simulink model "CVCA_TRAINING_21"  (R2021a)
settings: Solver=ode113  StartTime=0.0  StopTime=20  RelTol=1e-3
undefined symbols (not defined in the file or in its folder): Discrete, linsys1, Time
libraries: spsThreePhaseVIMeasurementLib x46, spsThreePhasePISectionLineLib x20, simulink x12, spsThreePhaseSeriesRLCLoadLib x12, spsThreePhaseBreakerLib x6, spsThreePhaseTransformerTwoWindingsLib x5, ctrlSharedLib x3, spsSynchronousMachinepuStandardLib x3, spsThreePhaseParallelRLCLoadLib x3, spsExcitationSystemLib x3, spsGenericPowerSystemStabilizerLib x3, spsHydraulicTurbineandGovernorLib x3
(part 1 of 2)
settings Model: Creator=root  LastModifiedBy=suman
settings DataIOCC: SaveFormat=Array  SaveOutput=off  SignalLogging=off  DSMLogging=off  SaveTime=off  ReturnWorkspaceOutputs=off
settings DebuggingCC: SFMachineParentedDataDiag=warning  ArithmeticOperatorsInVariantConditions=warning
settings SFSimCC: CustomCodeUndefinedFunction=UseInterfaceOnly

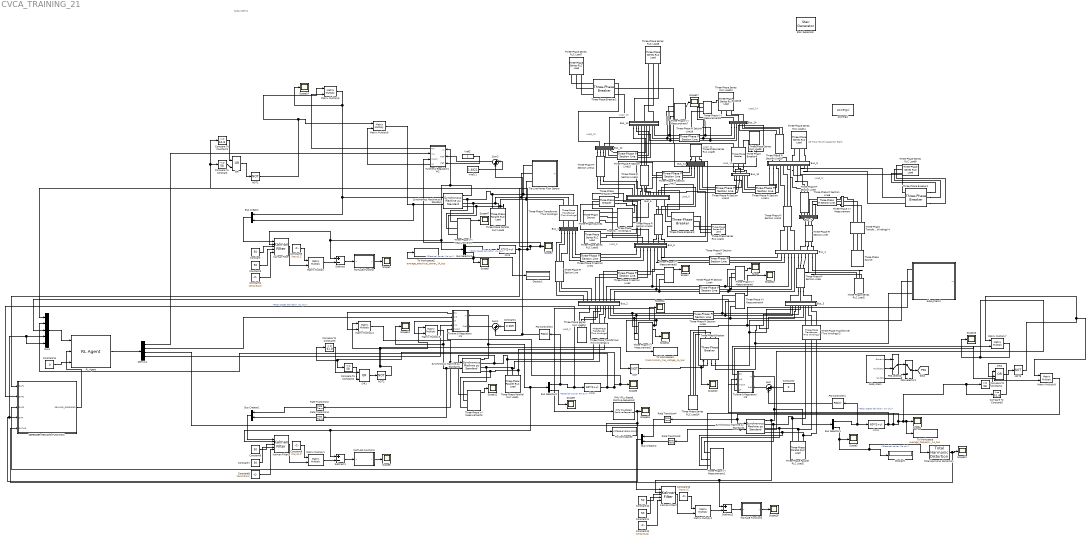
== system CVCA_TRAINING_21 ==
  note: Subsystem1
  note: Load_14
  note: Load_5
  note: Load_9
  note: Load_10
  note: 25 MVar Shunt
      | Capacitor Bank
  note: Load_6
  note: Load_11
  note: Load_13
  note: Load_12
  note: Load_2
  Bus Creator : BusCreator  Inputs=2
  Bus Creator1 : BusCreator  Inputs=2
  Bus Creator2 : BusCreator  Inputs=2
  Bus Selector1 : BusSelector  OutputSignals="Mechanical.Rotor speed deviation  dw (pu),Mechanical.Electrical power  Pe (pu)"
  Bus Selector2 : BusSelector  OutputSignals="Mechanical.Rotor speed deviation  dw (pu),Mechanical.Electrical power  Pe (pu)"
  Bus Selector3 : BusSelector  OutputSignals="Mechanical.Rotor speed deviation  dw (pu),Mechanical.Electrical power  Pe (pu)"
  Bus_1 : Subsystem
  Bus_10 : Subsystem
  Bus_11 : Subsystem
  Bus_12 : Subsystem
  Bus_13 : Subsystem
  Bus_14 : Subsystem
  Bus_2 : Subsystem
  Bus_3 : Subsystem
  Bus_4 : Subsystem
  Bus_5 : Subsystem
  Bus_6 : Subsystem
  Bus_7 : Subsystem
  Bus_9 : Subsystem
  Compare To Constant : simulink/Logic and Bit Operations/Compare To Constant  relop=<=  const=58  OutDataTypeStr=boolean
  Compare To Constant1 : simulink/Logic and Bit Operations/Compare To Constant  relop=>=  const=61.8  OutDataTypeStr=boolean
  Compare To Constant2 : simulink/Logic and Bit Operations/Compare To Constant  relop=<=  const=58  OutDataTypeStr=boolean
  Compare To Constant3 : simulink/Logic and Bit Operations/Compare To Constant  relop=>=  const=61.8  OutDataTypeStr=boolean
  Compare To Constant4 : simulink/Logic and Bit Operations/Compare To Constant  relop=<=  const=58  OutDataTypeStr=boolean
  Compare To Constant5 : simulink/Logic and Bit Operations/Compare To Constant  relop=>=  const=61.8  OutDataTypeStr=boolean
  Constant{,3,6..7,10..11} (6 alike) : Constant  Value=50
  Constant1 : Constant  Value=2.009
  Constant12 : Constant  Value=zeros(8,24)
  Constant13 : Constant  Value=linsys1.C
  Constant14 : Constant  Value=0
  Constant2 : Constant  Value=0
  Constant4 : Constant  Value=zeros(8,24)
  Constant5 : Constant  Value=linsys1.C
  Constant8 : Constant  Value=zeros(8,24)
  Constant9 : Constant  Value=linsys1.C
  DEFENDER REWARD FUNCTION : MATLAB Function  TreatAsAtomicUnit=on
  Demux1 : Demux
  Display1 : Display
  Display5 : Display
  Fcn1 : Fcn  Expr=60*(1+u)
  Fcn2 : Fcn  Expr=60*(1+u)
  Fcn3 : Fcn  Expr=60*(1+u)
  Kalman Filter : ctrlSharedLib/Kalman Filter  TimeDomain=Discrete-Time  UseCurrentEstimator=on  ModelSource=Individual A, B, C, D matrices  ModelSourceVariable=ss(0.95,1,1,0,1)  A=linsys1.A  B=linsys1.B  C=linsys1.C  D=linsys1.D  NumberOfStates=1  NumberOfInputs=1  NumberOfOutputs=1  InitialEstimateSource=Dialog  X0=0  P0=10  UseK=off  UseGH=off  NumberOfProcessNoiseInputs=1  G=1  TimeInvariantG=on  H=0  TimeInvariantH=on  Q=0.05  TimeInvariantQ=off  R=1  TimeInvariantR=off  N=0  TimeInvariantN=off  AddInputPort=on  AddEnablePort=off  OutputEstimatedY=off  OutputP=off  Ts=-1
  Kalman Filter1 : ctrlSharedLib/Kalman Filter  TimeDomain=Discrete-Time  UseCurrentEstimator=on  ModelSource=Individual A, B, C, D matrices  ModelSourceVariable=ss(0.95,1,1,0,1)  A=linsys1.A  B=linsys1.B  C=linsys1.C  D=linsys1.D  NumberOfStates=1  NumberOfInputs=1  NumberOfOutputs=1  InitialEstimateSource=Dialog  X0=0  P0=10  UseK=off  UseGH=off  NumberOfProcessNoiseInputs=1  G=1  TimeInvariantG=on  H=0  TimeInvariantH=on  Q=0.05  TimeInvariantQ=off  R=1  TimeInvariantR=off  N=0  TimeInvariantN=off  AddInputPort=on  AddEnablePort=off  OutputEstimatedY=off  OutputP=off  Ts=-1
  Kalman Filter2 : ctrlSharedLib/Kalman Filter  TimeDomain=Discrete-Time  UseCurrentEstimator=on  ModelSource=Individual A, B, C, D matrices  ModelSourceVariable=ss(0.95,1,1,0,1)  A=linsys1.A  B=linsys1.B  C=linsys1.C  D=linsys1.D  NumberOfStates=1  NumberOfInputs=1  NumberOfOutputs=1  InitialEstimateSource=Dialog  X0=0  P0=10  UseK=off  UseGH=off  NumberOfProcessNoiseInputs=1  G=1  TimeInvariantG=on  H=0  TimeInvariantH=on  Q=0.05  TimeInvariantQ=off  R=1  TimeInvariantR=off  N=0  TimeInvariantN=off  AddInputPort=on  AddEnablePort=off  OutputEstimatedY=off  OutputP=off  Ts=-1
  MATLAB Function : MATLAB Function  TreatAsAtomicUnit=on
  MATLAB Function1 : MATLAB Function  TreatAsAtomicUnit=on
  MATLAB Function2 : MATLAB Function  TreatAsAtomicUnit=on
  Matrix Multiply{,1..8} (9 alike) : Product  Multiplication=Matrix(*)
  Mux1 : Mux  Inputs=5
  NOT{,1..3} (4 alike) : Logic  Operator=NOT  IconShape=distinctive  AllPortsSameDT=off  OutDataTypeStr=boolean
  OR : Logic  Operator=OR  IconShape=distinctive  AllPortsSameDT=off  OutDataTypeStr=boolean
  OR1 : Logic  Operator=OR  IconShape=distinctive  AllPortsSameDT=off  OutDataTypeStr=boolean
  OR2 : Logic  Operator=OR  IconShape=distinctive  AllPortsSameDT=off  OutDataTypeStr=boolean
  PID Controller1 : slpidlib/PID Controller  Controller=PID  Form=Parallel  TimeDomain=Discrete-time  UseExternalTs=off  SampleTime=-1  IntegratorMethod=Forward Euler  FilterMethod=Forward Euler  ControllerParametersSource=internal  P=-0.020868  I=-0.0020766  D=0  UseFilter=on  N=100  TunerSelectOption=Frequency Response Based  InitialConditionSource=internal  InitialConditionForIntegrator=0  InitialConditionForFilter=0  DifferentiatorICPrevScaledInput=0  ExternalReset=none  TrackingMode=off  Kt=1  LimitOutput=off  SatLimitsSource=internal  UpperSaturationLimit=inf  LowerSaturationLimit=-inf  LinearizeAsGain=on  AntiWindupMode=none  Kb=1  POutMin=[]  POutMax=[]  IOutMin=[]  IOutMax=[]  DOutMin=[]  DOutMax=[]  NOutMin=[]  NOutMax=[]  SumOutMin=[]  SumOutMax=[]  SaturationOutMin=[]  SaturationOutMax=[]  PParamMin=[]  PParamMax=[]  IParamMin=[]  IParamMax=[]  DParamMin=[]  DParamMax=[]  NParamMin=[]  NParamMax=[]  KbParamMin=[]  KbParamMax=[]  KtParamMin=[]  KtParamMax=[]  KbOutMin=[]  KbOutMax=[]  KtOutMin=[]  KtOutMax=[]  IntegratorOutMin=[]  IntegratorOutMax=[]  FilterOutMin=[]  FilterOutMax=[]  SumI1OutMin=[]  SumI1OutMax=[]  SumI2OutMin=[]  SumI2OutMax=[]  SumI3OutMin=[]  SumI3OutMax=[]  SumI4OutMin=[]  SumI4OutMax=[]  SumDOutMin=[]  SumDOutMax=[]  DifferentiatorOutMin=[]  DifferentiatorOutMax=[]  FilterDiffOutCoefMin=[]  FilterDiffOutCoefMax=[]  ReciprocalOutMin=[]  ReciprocalOutMax=[]  SumDenOutMin=[]  SumDenOutMax=[]  SumNumOutMin=[]  SumNumOutMax=[]  DivideOutMin=[]  DivideOutMax=[]  UdiffTsProdOutMin=[]  UdiffTsProdOutMax=[]  NTsProdOutMin=[]  NTsProdOutMax=[]  UintegralTsProdOutMin=[]  UintegralTsProdOutMax=[]  UngainTsProdOutMin=[]  UngainTsProdOutMax=[]  IntegratorContinuousStateAttributes=''  IntegratorStateMustResolveToSignalObject=off  IntegratorRTWStateStorageClass=Auto  FilterContinuousStateAttributes=''  FilterStateMustResolveToSignalObject=off  FilterRTWStateStorageClass=Auto  ParallelPVariant=InternalParameters  IdealPVariant=Disabled  IVariant=InternalParameters  DVariant=InternalParameters  IntegratorVariant=Discrete  SatVariant=Disabled  AWVariant=Passthrough  PCopyVariant=Disabled  TRVariant=Disabled  FdbkBlocksVariant=Forward  IdealPFdbkVariant=Disabled  SatFdbkVariant=Disabled  DerivativeFilterVariant=ForwardEulerFilter  NVariant=InternalParameters  NCopyVariant=Disabled  FilterICVariant=InternalICsFilter  IntegratorICVariant=InternalICs  ExternalResetVariant=Disabled  TRSumVariant=Passthrough  SumFdbkVariant=Disabled  SumVariant=Sum_PID  TsampFilterVariant=InternalTs  TsampNgainVariant=Passthrough  TsampIntegralVariant=Passthrough  ExternalSaturationOutDataTypeStr=Inherit: Same as second input
  PID Controller2 : slpidlib/PID Controller  Controller=PID  Form=Parallel  TimeDomain=Discrete-time  UseExternalTs=off  SampleTime=-1  IntegratorMethod=Forward Euler  FilterMethod=Forward Euler  ControllerParametersSource=internal  P=-0.020868  I=-0.0020766  D=0  UseFilter=on  N=100  TunerSelectOption=Frequency Response Based  InitialConditionSource=internal  InitialConditionForIntegrator=0  InitialConditionForFilter=0  DifferentiatorICPrevScaledInput=0  ExternalReset=none  TrackingMode=off  Kt=1  LimitOutput=off  SatLimitsSource=internal  UpperSaturationLimit=inf  LowerSaturationLimit=-inf  LinearizeAsGain=on  AntiWindupMode=none  Kb=1  POutMin=[]  POutMax=[]  IOutMin=[]  IOutMax=[]  DOutMin=[]  DOutMax=[]  NOutMin=[]  NOutMax=[]  SumOutMin=[]  SumOutMax=[]  SaturationOutMin=[]  SaturationOutMax=[]  PParamMin=[]  PParamMax=[]  IParamMin=[]  IParamMax=[]  DParamMin=[]  DParamMax=[]  NParamMin=[]  NParamMax=[]  KbParamMin=[]  KbParamMax=[]  KtParamMin=[]  KtParamMax=[]  KbOutMin=[]  KbOutMax=[]  KtOutMin=[]  KtOutMax=[]  IntegratorOutMin=[]  IntegratorOutMax=[]  FilterOutMin=[]  FilterOutMax=[]  SumI1OutMin=[]  SumI1OutMax=[]  SumI2OutMin=[]  SumI2OutMax=[]  SumI3OutMin=[]  SumI3OutMax=[]  SumI4OutMin=[]  SumI4OutMax=[]  SumDOutMin=[]  SumDOutMax=[]  DifferentiatorOutMin=[]  DifferentiatorOutMax=[]  FilterDiffOutCoefMin=[]  FilterDiffOutCoefMax=[]  ReciprocalOutMin=[]  ReciprocalOutMax=[]  SumDenOutMin=[]  SumDenOutMax=[]  SumNumOutMin=[]  SumNumOutMax=[]  DivideOutMin=[]  DivideOutMax=[]  UdiffTsProdOutMin=[]  UdiffTsProdOutMax=[]  NTsProdOutMin=[]  NTsProdOutMax=[]  UintegralTsProdOutMin=[]  UintegralTsProdOutMax=[]  UngainTsProdOutMin=[]  UngainTsProdOutMax=[]  IntegratorContinuousStateAttributes=''  IntegratorStateMustResolveToSignalObject=off  IntegratorRTWStateStorageClass=Auto  FilterContinuousStateAttributes=''  FilterStateMustResolveToSignalObject=off  FilterRTWStateStorageClass=Auto  ParallelPVariant=InternalParameters  IdealPVariant=Disabled  IVariant=InternalParameters  DVariant=InternalParameters  IntegratorVariant=Discrete  SatVariant=Disabled  AWVariant=Passthrough  PCopyVariant=Disabled  TRVariant=Disabled  FdbkBlocksVariant=Forward  IdealPFdbkVariant=Disabled  SatFdbkVariant=Disabled  DerivativeFilterVariant=ForwardEulerFilter  NVariant=InternalParameters  NCopyVariant=Disabled  FilterICVariant=InternalICsFilter  IntegratorICVariant=InternalICs  ExternalResetVariant=Disabled  TRSumVariant=Passthrough  SumFdbkVariant=Disabled  SumVariant=Sum_PID  TsampFilterVariant=InternalTs  TsampNgainVariant=Passthrough  TsampIntegralVariant=Passthrough  ExternalSaturationOutDataTypeStr=Inherit: Same as second input
  "PMU (PLL-Based, Positive-Sequence)" : spsPMUPLLBasedPositiveSequenceLib/PMU (PLL-Based, Positive-Sequence)  nominalFrequency=60  samplingRate=64  reportingFactor=1
      settings: SourceProductBaseCode=PS
  PSS selector : ManualSwitch  CurrentSetting=0
  PSS selector1 : ManualSwitch
  RL Agent : rllib/RL Agent  Agent=agentCVCA_21  ExternalActionAsInput=off  ProvideCumRwd=off  TreatAsDirectFeedthrough=on
  Rate Transition{2..5} (4 alike) : RateTransition
  Scope{,1..21,24,47} (24 alike) : Scope
  Stair Generator : eeStairGenerator/Stair Generator  LabelModeActiveChoice=Discrete  TimeInput=[1 2 3 4 5 6 7 8 9 10]  AmplitudeInput=[0 1 0 1 0 1 0 1 0 1]  SampleTime=1  RepeatPattern=off  OutDataTypeStr=double
      settings: SourceProductBaseCode=PS
  Subsystem : Subsystem
  Subsystem2 : Subsystem
      mask Display: image('C:\Users\suman\Downloads\Gridsense-Line-IQ-Advanced-Distribution-Submission-Line-Monitoring-2.jpg'); % Use "Edit Image" on toolstrip to change.
  Subtract : Sum  Inputs=+-
  Subtract1 : Sum  Inputs=+-
  Subtract2 : Sum  Inputs=+-
  Sum : Sum  Inputs=|++
  Sum1 : Sum  Inputs=|++
  Sum2 : Sum  Inputs=|++
  Synchronous Machine pu Standard : spsSynchronousMachinepuStandardLib/Synchronous Machine pu Standard  PresetModel=No  MechanicalLoad=Mechanical power Pm  ShowDetailedParameters=on  RotorType=Salient-pole  Units=per unit standard parameters  MeasurementBus=off  NominalParameters="[90E6  146280   60 ]"  Reactances1=[ 1.81, 0.3, 0.23, 1.76, 0.65, 0.25, 0.15 ]  Reactances2=[ 1.305, 0.296, 0.252, 0.474, 0.243, 0.18 ]  dAxisTimeConstants=Short-circuit  qAxisTimeConstants=Open-circuit  TimeConstants1="[ 4.4849  0.0681  0.1  ]"  TimeConstants2=[ 8.0, 0.03, 1.0, 0.07 ]  TimeConstants3="[  4.49  0.0681  0.0513  ]"  TimeConstants4=[ 8.0, 0.03, 0.3371, 0.0295 ]  TimeConstants5=[ 1.01, 0.053, 0.1 ]  TimeConstants6=[ 1.3201, 0.023, 1.0, 0.07 ]  TimeConstants7=[0.012 0.003 0.003]  TimeConstants8=[ 1.3201, 0.0231, 0.3371, 0.0295 ]  StatorResistance=2.8544e-3  Mechanical="[ 3.7 0  32]"  PolePairs=20  InitialConditions=[0 -55.1684 1.72023 1.72023 1.72023 -10.3587 -130.359 109.641 2.41694]  SetSaturation=off  Saturation=[0.6404,0.7127,0.8441,0.9214,0.9956,1.082,1.19,1.316,1.457;0.7,0.7698,0.8872,0.9466,0.9969,1.046,1.1,1.151,1.201]  LoadFlowParameters=[1 0 0 0 0]  TsPowergui=0  TsBlock=-1  IterativeModel=Trapezoidal non iterative  IterativeDiscreteModel=Trapezoidal non iterative  BusType=swing  Pref=0  Qref=0  Qmin=-inf  Qmax=inf  PLF=0  QLF=0
      settings: SourceProductBaseCode=PS
  Synchronous Machine pu Standard1 : spsSynchronousMachinepuStandardLib/Synchronous Machine pu Standard  PresetModel=No  MechanicalLoad=Mechanical power Pm  ShowDetailedParameters=on  RotorType=Salient-pole  Units=per unit standard parameters  MeasurementBus=off  NominalParameters="[90E6  144210   60 ]"  Reactances1=[ 1.81, 0.3, 0.23, 1.76, 0.65, 0.25, 0.15 ]  Reactances2=[ 1.305, 0.296, 0.252, 0.474, 0.243, 0.18 ]  dAxisTimeConstants=Short-circuit  qAxisTimeConstants=Open-circuit  TimeConstants1="[ 4.4849  0.0681  0.1  ]"  TimeConstants2=[ 8.0, 0.03, 1.0, 0.07 ]  TimeConstants3="[  4.49  0.0681  0.0513  ]"  TimeConstants4=[ 8.0, 0.03, 0.3371, 0.0295 ]  TimeConstants5=[ 1.01, 0.053, 0.1 ]  TimeConstants6=[ 1.3201, 0.023, 1.0, 0.07 ]  TimeConstants7=[0.012 0.003 0.003]  TimeConstants8=[ 1.3201, 0.0231, 0.3371, 0.0295 ]  StatorResistance=2.8544e-3  Mechanical="[ 3.7 0  32]"  PolePairs=20  InitialConditions=[0 -52.2742 2.06355 2.06355 2.06355 -13.2061 -133.206 106.794 2.88545]  SetSaturation=off  Saturation=[0.6404,0.7127,0.8441,0.9214,0.9956,1.082,1.19,1.316,1.457;0.7,0.7698,0.8872,0.9466,0.9969,1.046,1.1,1.151,1.201]  LoadFlowParameters=[1,0,0,0,0]  TsPowergui=0  TsBlock=-1  IterativeModel=Trapezoidal non iterative  IterativeDiscreteModel=Trapezoidal non iterative  BusType=PV  Pref=0  Qref=0  Qmin=-inf  Qmax=inf  PLF=0  QLF=0
      settings: SourceProductBaseCode=PS
  Synchronous Machine pu Standard2 : spsSynchronousMachinepuStandardLib/Synchronous Machine pu Standard  PresetModel=No  MechanicalLoad=Mechanical power Pm  ShowDetailedParameters=on  RotorType=Salient-pole  Units=per unit standard parameters  MeasurementBus=off  NominalParameters="[90E6  139380  60 ]"  Reactances1=[ 1.81, 0.3, 0.23, 1.76, 0.65, 0.25, 0.15 ]  Reactances2=[ 1.305, 0.296, 0.252, 0.474, 0.243, 0.18 ]  dAxisTimeConstants=Short-circuit  qAxisTimeConstants=Open-circuit  TimeConstants1="[ 4.4849  0.0681  0.1  ]"  TimeConstants2=[ 8.0, 0.03, 1.0, 0.07 ]  TimeConstants3="[  4.49  0.0681  0.0513  ]"  TimeConstants4=[ 8.0, 0.03, 0.3371, 0.0295 ]  TimeConstants5=[ 1.01, 0.053, 0.1 ]  TimeConstants6=[ 1.3201, 0.023, 1.0, 0.07 ]  TimeConstants7=[0.012 0.003 0.003]  TimeConstants8=[ 1.3201, 0.0231, 0.3371, 0.0295 ]  StatorResistance=2.8544e-3  Mechanical="[ 3.7 0  32]"  PolePairs=20  InitialConditions=[0 -114.329 0.550177 0.550177 0.550177 -114.259 -234.259 5.74123 1.7297]  SetSaturation=off  Saturation=[0.6404,0.7127,0.8441,0.9214,0.9956,1.082,1.19,1.316,1.457;0.7,0.7698,0.8872,0.9466,0.9969,1.046,1.1,1.151,1.201]  LoadFlowParameters=[1,0,0,0,0]  TsPowergui=0  TsBlock=-1  IterativeModel=Trapezoidal non iterative  IterativeDiscreteModel=Trapezoidal non iterative  BusType=PV  Pref=0  Qref=0  Qmin=50096006  Qmax=50096006  PLF=0  QLF=0
      settings: SourceProductBaseCode=PS
  Three-Phase PI Section Line : spsThreePhasePISectionLineLib/Three-Phase PI Section Line  LConnTagsString=a|b|c  RConnTagsString=A|B|C  Length=44.47  Frequency=60  Resistances=[ 0.1921 0.5763]  Inductances=[ 0.0016 0.0047]  Capacitances=[7.14e-9 2.14e-8]
  Three-Phase PI Section Line1 : spsThreePhasePISectionLineLib/Three-Phase PI Section Line  LConnTagsString=a|b|c  RConnTagsString=A|B|C  Length=78.64  Frequency=60  Resistances=[ 0.3029 0.9086]  Inductances=[ 0.0033 0.0099]  Capacitances=[3.35e-9 1.01e-8]
  Three-Phase PI Section Line10 : spsThreePhasePISectionLineLib/Three-Phase PI Section Line  LConnTagsString=a|b|c  RConnTagsString=A|B|C  Length=8.39  Frequency=60  Resistances=[ 0.0001 0.0003]  Inductances=[ 0.0775 0.2325]  Capacitances=[1.43e-10 4.3e-10]
  Three-Phase PI Section Line11 : spsThreePhasePISectionLineLib/Three-Phase PI Section Line  LConnTagsString=a|b|c  RConnTagsString=A|B|C  Length=3.27  Frequency=60  Resistances=[ 0.2144 0.6431]  Inductances=[ 0.0015 0.0045]  Capacitances=[1.84e-11 5.52e-11]
  Three-Phase PI Section Line12 : spsThreePhasePISectionLineLib/Three-Phase PI Section Line  LConnTagsString=a|b|c  RConnTagsString=A|B|C  Length=4.93  Frequency=60  Resistances=[ 0.3667 1.1002]  Inductances=[ 0.0023 0.0068]  Capacitances=[1.22e-11 3.66e-11]
  Three-Phase PI Section Line13 : spsThreePhasePISectionLineLib/Three-Phase PI Section Line  LConnTagsString=a|b|c  RConnTagsString=A|B|C  Length=5.65  Frequency=60  Resistances=[ 0.0001 0.0003]  Inductances=[ 0.0522 0.1565]  Capacitances=[2.13e-10 6.39e-10]
  Three-Phase PI Section Line14 : spsThreePhasePISectionLineLib/Three-Phase PI Section Line  LConnTagsString=a|b|c  RConnTagsString=A|B|C  Length=5.69  Frequency=60  Resistances=[ 0.4760 1.4281]  Inductances=[ 0.0026 0.0079]  Capacitances=[1.06e-11 3.17e-11]
  Three-Phase PI Section Line15 : spsThreePhasePISectionLineLib/Three-Phase PI Section Line  LConnTagsString=a|b|c  RConnTagsString=A|B|C  Length=5.03  Frequency=60  Resistances=[ 0.9679 2.9038]  Inductances=[ 0.0023 0.0070]  Capacitances=[1.20e-11 3.59e-11]
  Three-Phase PI Section Line16 : spsThreePhasePISectionLineLib/Three-Phase PI Section Line  LConnTagsString=a|b|c  RConnTagsString=A|B|C  Length=4.06  Frequency=60  Resistances=[ 0.3590 1.0770]  Inductances=[ 0.0019 0.0056]  Capacitances=[1.48e-11 4.44e-11]
  Three-Phase PI Section Line17 : spsThreePhasePISectionLineLib/Three-Phase PI Section Line  LConnTagsString=a|b|c  RConnTagsString=A|B|C  Length=5.02  Frequency=60  Resistances=[ 0.4172 1.2515]  Inductances=[ 0.0023 0.0070]  Capacitances=[1.20e-11 3.60e-11]
  Three-Phase PI Section Line18 : spsThreePhasePISectionLineLib/Three-Phase PI Section Line  LConnTagsString=a|b|c  RConnTagsString=A|B|C  Length=6.64  Frequency=60  Resistances=[ 0.5676 1.7027]  Inductances=[ 0.0031 0.0092]  Capacitances=[9.06e-12 2.72e-11]
  Three-Phase PI Section Line19 : spsThreePhasePISectionLineLib/Three-Phase PI Section Line  LConnTagsString=a|b|c  RConnTagsString=A|B|C  Length=5.85  Frequency=60  Resistances=[ 0.4788 1.4365]  Inductances=[ 0.0027 0.0081]  Capacitances=[1.03e-11 3.08e-11]
  Three-Phase PI Section Line2 : spsThreePhasePISectionLineLib/Three-Phase PI Section Line  LConnTagsString=a|b|c  RConnTagsString=A|B|C  Length=61.18  Frequency=60  Resistances=[ 0.4104 1.2311]  Inductances=[ 0.0033 0.0100]  Capacitances=[3.34e-9 1.0e-8]
  Three-Phase PI Section Line3 : spsThreePhasePISectionLineLib/Three-Phase PI Section Line  LConnTagsString=a|b|c  RConnTagsString=A|B|C  Length=18.47  Frequency=60  Resistances=[ 0.3186 0.9558]  Inductances=[ 0.0027 0.0080]  Capacitances=[4.17e-9 1.25e-8]
  Three-Phase PI Section Line4 : spsThreePhasePISectionLineLib/Three-Phase PI Section Line  LConnTagsString=a|b|c  RConnTagsString=A|B|C  Length=74.11  Frequency=60  Resistances=[ 0.3457 1.0370]  Inductances=[ 0.0028 0.0083]  Capacitances=[3.99e-9 1.20e-8]
  Three-Phase PI Section Line5 : spsThreePhasePISectionLineLib/Three-Phase PI Section Line  LConnTagsString=a|b|c  RConnTagsString=A|B|C  Length=68.47  Frequency=60  Resistances=[ 0.3026 0.9077]  Inductances=[ 0.0034 0.0101]  Capacitances=[3.29e-9 9.86e-8]
  Three-Phase PI Section Line6 : spsThreePhasePISectionLineLib/Three-Phase PI Section Line  LConnTagsString=a|b|c  RConnTagsString=A|B|C  Length=61.21  Frequency=60  Resistances=[ 0.4826 1.4479]  Inductances=[ 0.0033 0.0098]  Capacitances=[3.4e-9 1.02e-8]
  Three-Phase PI Section Line7 : spsThreePhasePISectionLineLib/Three-Phase PI Section Line  LConnTagsString=a|b|c  RConnTagsString=A|B|C  Length=5.15  Frequency=60  Resistances=[ 0.0001 0.0003]  Inductances=[ 0.0475 0.1425]  Capacitances=[2.34e-10 7.02e-10]
  Three-Phase PI Section Line8 : spsThreePhasePISectionLineLib/Three-Phase PI Section Line  LConnTagsString=a|b|c  RConnTagsString=A|B|C  Length=4.72  Frequency=60  Resistances=[ 0.0005 0.0014]  Inductances=[ 0.0022 0.0065]  Capacitances=[ 1.27e-11 3.82e-11]
  Three-Phase PI Section Line9 : spsThreePhasePISectionLineLib/Three-Phase PI Section Line  LConnTagsString=a|b|c  RConnTagsString=A|B|C  Length=3.73  Frequency=60  Resistances=[ 0.0006 0.0018]  Inductances=[ 0.0017 0.0052]  Capacitances=[ 1.61e-11 4.84e-11]
  Three-Phase Parallel RLC Load1 : spsThreePhaseParallelRLCLoadLib/Three-Phase Parallel RLC Load  LConnTagsString=A|B|C  Configuration=Y (grounded)  NominalVoltage=10000  Vabc=[1e3 1e3 1e3]  Vabcp=[1e3 1e3 1e3]  NominalFrequency=60  UnbalancedPower=off  ActivePower=10e3  InductivePower=2000  CapacitivePower=0  Pabc=[10e3 9e3 11e3]  QLabc=[100 90 110]  QCabc=[100 90 110]  Pabcp=[10e3 9e3 11e3]  QLabcp=[100 90 110]  QCabcp=[100 90 110]  Measurements=None  LoadType=constant Z
  Three-Phase Parallel RLC Load2 : spsThreePhaseParallelRLCLoadLib/Three-Phase Parallel RLC Load  LConnTagsString=A|B|C  Configuration=Y (grounded)  NominalVoltage=10000  Vabc=[1e3 1e3 1e3]  Vabcp=[1e3 1e3 1e3]  NominalFrequency=60  UnbalancedPower=off  ActivePower=10e3  InductivePower=2000  CapacitivePower=0  Pabc=[10e3 9e3 11e3]  QLabc=[100 90 110]  QCabc=[100 90 110]  Pabcp=[10e3 9e3 11e3]  QLabcp=[100 90 110]  QCabcp=[100 90 110]  Measurements=None  LoadType=constant Z
  Three-Phase Parallel RLC Load3 : spsThreePhaseParallelRLCLoadLib/Three-Phase Parallel RLC Load  LConnTagsString=A|B|C  Configuration=Y (grounded)  NominalVoltage=10000  Vabc=[1e3 1e3 1e3]  Vabcp=[1e3 1e3 1e3]  NominalFrequency=60  UnbalancedPower=off  ActivePower=10e3  InductivePower=2000  CapacitivePower=0  Pabc=[10e3 9e3 11e3]  QLabc=[100 90 110]  QCabc=[100 90 110]  Pabcp=[10e3 9e3 11e3]  QLabcp=[100 90 110]  QCabcp=[100 90 110]  Measurements=None  LoadType=constant Z
  Three-Phase Series RLC Load10 : spsThreePhaseSeriesRLCLoadLib/Three-Phase Series RLC Load  LConnTagsString=A|B|C  Configuration=Y (grounded)  NominalVoltage=(222552)*1  Vabc=[1e3 1e3 1e3]  Vabcp=[1e3 1e3 1e3]  NominalFrequency=60  UnbalancedPower=off  ActivePower=26040000  InductivePower=15240000  CapacitivePower=0  Pabc=[10e3 9e3 11e3]  QLabc=[100 90 110]  QCabc=[100 90 110]  Pabcp=[10e3 9e3 11e3]  QLabcp=[100 90 110]  QCabcp=[100 90 110]  Measurements=None  LoadType=constant PQ
  Three-Phase Series RLC Load11 : spsThreePhaseSeriesRLCLoadLib/Three-Phase Series RLC Load  LConnTagsString=A|B|C  Configuration=Y (grounded)  NominalVoltage=230e3  Vabc=[1e3 1e3 1e3]  Vabcp=[1e3 1e3 1e3]  NominalFrequency=60  UnbalancedPower=off  ActivePower=0  InductivePower=0  CapacitivePower=2500000000  Pabc=[10e3 9e3 11e3]  QLabc=[100 90 110]  QCabc=[100 90 110]  Pabcp=[10e3 9e3 11e3]  QLabcp=[100 90 110]  QCabcp=[100 90 110]  Measurements=None  LoadType=constant Z
  Three-Phase Series RLC Load12 : spsThreePhaseSeriesRLCLoadLib/Three-Phase Series RLC Load  LConnTagsString=A|B|C  Configuration=Y (grounded)  NominalVoltage=(221100)*1  Vabc=[1e3 1e3 1e3]  Vabcp=[1e3 1e3 1e3]  NominalFrequency=60  UnbalancedPower=off  ActivePower=17880000  InductivePower=6000000  CapacitivePower=0  Pabc=[10e3 9e3 11e3]  QLabc=[100 90 110]  QCabc=[100 90 110]  Pabcp=[10e3 9e3 11e3]  QLabcp=[100 90 110]  QCabcp=[100 90 110]  Measurements=None  LoadType=constant PQ
  Three-Phase Series RLC Load14 : spsThreePhaseSeriesRLCLoadLib/Three-Phase Series RLC Load  LConnTagsString=A|B|C  Configuration=Y (grounded)  NominalVoltage=(217684)*1  Vabc=[1e3 1e3 1e3]  Vabcp=[1e3 1e3 1e3]  NominalFrequency=60  UnbalancedPower=off  ActivePower=1130400000000  InductivePower=228000000000  CapacitivePower=0  Pabc=[10e3 9e3 11e3]  QLabc=[100 90 110]  QCabc=[100 90 110]  Pabcp=[10e3 9e3 11e3]  QLabcp=[100 90 110]  QCabcp=[100 90 110]  Measurements=None  LoadType=constant PQ
  Three-Phase Series RLC Load2 : spsThreePhaseSeriesRLCLoadLib/Three-Phase Series RLC Load  LConnTagsString=A|B|C  Configuration=Y (grounded)  NominalVoltage=(217810)*1  Vabc=[1e3 1e3 1e3]  Vabcp=[1e3 1e3 1e3]  NominalFrequency=60  UnbalancedPower=off  ActivePower=57360000  InductivePower=0  CapacitivePower=4680000  Pabc=[10e3 9e3 11e3]  QLabc=[100 90 110]  QCabc=[100 90 110]  Pabcp=[10e3 9e3 11e3]  QLabcp=[100 90 110]  QCabcp=[100 90 110]  Measurements=None  LoadType=constant PQ
  Three-Phase Series RLC Load3 : spsThreePhaseSeriesRLCLoadLib/Three-Phase Series RLC Load  LConnTagsString=A|B|C  Configuration=Y (grounded)  NominalVoltage=(218590)*1  Vabc=[1e3 1e3 1e3]  Vabcp=[1e3 1e3 1e3]  NominalFrequency=60  UnbalancedPower=off  ActivePower=9120000  InductivePower=1920000  CapacitivePower=0  Pabc=[10e3 9e3 11e3]  QLabc=[100 90 110]  QCabc=[100 90 110]  Pabcp=[10e3 9e3 11e3]  QLabcp=[100 90 110]  QCabcp=[100 90 110]  Measurements=None  LoadType=constant PQ
  Three-Phase Series RLC Load4 : spsThreePhaseSeriesRLCLoadLib/Three-Phase Series RLC Load  LConnTagsString=A|B|C  Configuration=Y (grounded)  NominalVoltage=(221344)*1.00001  Vabc=[1e3 1e3 1e3]  Vabcp=[1e3 1e3 1e3]  NominalFrequency=60  UnbalancedPower=off  ActivePower=13440000  InductivePower=9000000  CapacitivePower=0  Pabc=[10e3 9e3 11e3]  QLabc=[100 90 110]  QCabc=[100 90 110]  Pabcp=[10e3 9e3 11e3]  QLabcp=[100 90 110]  QCabcp=[100 90 110]  Measurements=None  LoadType=constant PQ
  Three-Phase Series RLC Load5 : spsThreePhaseSeriesRLCLoadLib/Three-Phase Series RLC Load  LConnTagsString=A|B|C  Configuration=Y (grounded)  NominalVoltage=(221346)*1  Vabc=[1e3 1e3 1e3]  Vabcp=[1e3 1e3 1e3]  NominalFrequency=60  UnbalancedPower=off  ActivePower=10800  InductivePower=6960000  CapacitivePower=0  Pabc=[10e3 9e3 11e3]  QLabc=[100 90 110]  QCabc=[100 90 110]  Pabcp=[10e3 9e3 11e3]  QLabcp=[100 90 110]  QCabcp=[100 90 110]  Measurements=None  LoadType=constant PQ
  Three-Phase Series RLC Load6 : spsThreePhaseSeriesRLCLoadLib/Three-Phase Series RLC Load  LConnTagsString=A|B|C  Configuration=Y (grounded)  NominalVoltage=(221304)*1  Vabc=[1e3 1e3 1e3]  Vabcp=[1e3 1e3 1e3]  NominalFrequency=60  UnbalancedPower=off  ActivePower=4200000  InductivePower=2160000  CapacitivePower=0  Pabc=[10e3 9e3 11e3]  QLabc=[100 90 110]  QCabc=[100 90 110]  Pabcp=[10e3 9e3 11e3]  QLabcp=[100 90 110]  QCabcp=[100 90 110]  Measurements=None  LoadType=constant PQ
  Three-Phase Series RLC Load7 : spsThreePhaseSeriesRLCLoadLib/Three-Phase Series RLC Load  LConnTagsString=A|B|C  Configuration=Y (grounded)  NominalVoltage=(221181)*1  Vabc=[1e3 1e3 1e3]  Vabcp=[1e3 1e3 1e3]  NominalFrequency=60  UnbalancedPower=off  ActivePower=7320000  InductivePower=1920000  CapacitivePower=0  Pabc=[10e3 9e3 11e3]  QLabc=[100 90 110]  QCabc=[100 90 110]  Pabcp=[10e3 9e3 11e3]  QLabcp=[100 90 110]  QCabcp=[100 90 110]  Measurements=None  LoadType=constant PQ
  Three-Phase Series RLC Load8 : spsThreePhaseSeriesRLCLoadLib/Three-Phase Series RLC Load  LConnTagsString=A|B|C  Configuration=Y (grounded)  NominalVoltage=(221144)*0.999998  Vabc=[1e3 1e3 1e3]  Vabcp=[1e3 1e3 1e3]  NominalFrequency=60  UnbalancedPower=off  ActivePower=1620000  InductivePower=6960000  CapacitivePower=0  Pabc=[10e3 9e3 11e3]  QLabc=[100 90 110]  QCabc=[100 90 110]  Pabcp=[10e3 9e3 11e3]  QLabcp=[100 90 110]  QCabcp=[100 90 110]  Measurements=None  LoadType=constant PQ
  Three-Phase Series RLC Load9 : spsThreePhaseSeriesRLCLoadLib/Three-Phase Series RLC Load  LConnTagsString=A|B|C  Configuration=Y (grounded)  NominalVoltage=(221458)*1  Vabc=[1e3 1e3 1e3]  Vabcp=[1e3 1e3 1e3]  NominalFrequency=60  UnbalancedPower=off  ActivePower=35400000  InductivePower=19920000  CapacitivePower=0  Pabc=[10e3 9e3 11e3]  QLabc=[100 90 110]  QCabc=[100 90 110]  Pabcp=[10e3 9e3 11e3]  QLabcp=[100 90 110]  QCabcp=[100 90 110]  Measurements=None  LoadType=constant PQ
  Three-Phase Transformer (Two Windings) : spsThreePhaseTransformerTwoWindingsLib/Three-Phase Transformer (Two Windings)  Winding1Connection=Yg  Winding2Connection=Yg  CoreType=Three single-phase transformers  SetSaturation=off  Hysteresis=off  DataFile='hysteresis'  SetInitialFlux=off  Measurements=None  UNITS=pu  NominalPower=[ 120e6 , 60 ]  Winding1=[146.28e3 , 0.002 , 0.08 ]  Winding2=[ 230e3 , 0.002 , 0.08 ]  Rm=500  Lm=500  L0=0.5  Saturation=[ 0,0 ; 0.0024,1.2 ; 1.0,1.52 ]  InitialFluxes=[ 0.8 , -0.8 , 0.7 ]  BreakLoop=off  DiscreteSolver=Trapezoidal iterative  DataType=off  TransfoNumber=1
  Three-Phase Transformer (Two Windings)1 : spsThreePhaseTransformerTwoWindingsLib/Three-Phase Transformer (Two Windings)  Winding1Connection=Yg  Winding2Connection=Yg  CoreType=Three single-phase transformers  SetSaturation=off  Hysteresis=off  DataFile='hysteresis'  SetInitialFlux=off  Measurements=None  UNITS=pu  NominalPower=[ 120e6 , 60 ]  Winding1=[144.21e3 , 0.002 , 0.08 ]  Winding2=[ 230e3 , 0.002 , 0.08 ]  Rm=500  Lm=500  L0=0.5  Saturation=[ 0,0 ; 0.0024,1.2 ; 1.0,1.52 ]  InitialFluxes=[ 0.8 , -0.8 , 0.7 ]  BreakLoop=off  DiscreteSolver=Trapezoidal iterative  DataType=off  TransfoNumber=1
  Three-Phase Transformer (Two Windings)2 : spsThreePhaseTransformerTwoWindingsLib/Three-Phase Transformer (Two Windings)  Winding1Connection=Yg  Winding2Connection=Yg  CoreType=Three single-phase transformers  SetSaturation=off  Hysteresis=off  DataFile='hysteresis'  SetInitialFlux=off  Measurements=None  UNITS=pu  NominalPower=[ 120e6 , 60 ]  Winding1=[147.66e3 , 0.002 , 0.08 ]  Winding2=[ 230e3 , 0.002 , 0.08 ]  Rm=500  Lm=500  L0=0.5  Saturation=[ 0,0 ; 0.0024,1.2 ; 1.0,1.52 ]  InitialFluxes=[ 0.8 , -0.8 , 0.7 ]  BreakLoop=off  DiscreteSolver=Trapezoidal iterative  DataType=off  TransfoNumber=1
  Three-Phase Transformer (Two Windings)3 : spsThreePhaseTransformerTwoWindingsLib/Three-Phase Transformer (Two Windings)  Winding1Connection=Yg  Winding2Connection=Yg  CoreType=Three single-phase transformers  SetSaturation=off  Hysteresis=off  DataFile='hysteresis'  SetInitialFlux=off  Measurements=None  UNITS=pu  NominalPower=[ 120e6 , 60 ]  Winding1=[139.38e3 , 0.002 , 0.08 ]  Winding2=[ 230e3 , 0.002 , 0.08 ]  Rm=500  Lm=500  L0=0.5  Saturation=[ 0,0 ; 0.0024,1.2 ; 1.0,1.52 ]  InitialFluxes=[ 0.8 , -0.8 , 0.7 ]  BreakLoop=off  DiscreteSolver=Trapezoidal iterative  DataType=off  TransfoNumber=1
  Three-Phase Transformer (Two Windings)4 : spsThreePhaseTransformerTwoWindingsLib/Three-Phase Transformer (Two Windings)  Winding1Connection=Yg  Winding2Connection=Yg  CoreType=Three single-phase transformers  SetSaturation=off  Hysteresis=off  DataFile='hysteresis'  SetInitialFlux=off  Measurements=None  UNITS=pu  NominalPower=[ 120e6 , 60 ]  Winding1=[150.42e3 , 0.002 , 0.08 ]  Winding2=[ 230e3 , 0.002 , 0.08 ]  Rm=500  Lm=500  L0=0.5  Saturation=[ 0,0 ; 0.0024,1.2 ; 1.0,1.52 ]  InitialFluxes=[ 0.8 , -0.8 , 0.7 ]  BreakLoop=off  DiscreteSolver=Trapezoidal iterative  DataType=off  TransfoNumber=1
  Three-Phase V-I Measurement : spsThreePhaseVIMeasurementLib/Three-Phase V-I Measurement  VoltageMeasurement=phase-to-phase  SetLabelV=on  LabelV=VB_8  Vpu=off  VpuLL=off  CurrentMeasurement=yes  SetLabelI=on  LabelI=IB_8  Ipu=off  Pbase=100e6  Vbase=500e3  OutputType=Complex  PhasorSimulation=off  PSBequivalent=0
  Three-Phase V-I Measurement{1..9} (9 alike) : spsThreePhaseVIMeasurementLib/Three-Phase V-I Measurement  VoltageMeasurement=phase-to-ground  SetLabelV=off  LabelV=Vabc  Vpu=off  VpuLL=off  CurrentMeasurement=yes  SetLabelI=off  LabelI=Iabc  Ipu=off  Pbase=100e6  Vbase=500e3  OutputType=Complex  PhasorSimulation=off  PSBequivalent=0
  Three-Phase Breaker : spsThreePhaseBreakerLib/Three-Phase Breaker  InitialState=open  SwitchA=on  SwitchB=on  SwitchC=on  SwitchTimes="[1/60  5/60]"  External=on  BreakerResistance=0.00001  SnubberResistance=1e16  SnubberCapacitance=inf  Measurements=None
  Three-Phase Breaker1 : spsThreePhaseBreakerLib/Three-Phase Breaker  InitialState=closed  SwitchA=on  SwitchB=on  SwitchC=on  SwitchTimes=[10000000000]  External=off  BreakerResistance=0.00001  SnubberResistance=1e16  SnubberCapacitance=inf  Measurements=None
  Three-Phase Breaker2 : spsThreePhaseBreakerLib/Three-Phase Breaker  InitialState=closed  SwitchA=on  SwitchB=on  SwitchC=on  SwitchTimes=[10000000000]  External=off  BreakerResistance=0.0001  SnubberResistance=1e16  SnubberCapacitance=inf  Measurements=None
  Three-Phase Breaker3 : spsThreePhaseBreakerLib/Three-Phase Breaker  InitialState=closed  SwitchA=on  SwitchB=on  SwitchC=on  SwitchTimes=[10000000000]  External=off  BreakerResistance=0.0001  SnubberResistance=1e16  SnubberCapacitance=inf  Measurements=None
  Three-Phase Breaker4 : spsThreePhaseBreakerLib/Three-Phase Breaker  InitialState=open  SwitchA=on  SwitchB=on  SwitchC=on  SwitchTimes="[1/60  5/60]"  External=on  BreakerResistance=0.0001  SnubberResistance=1e16  SnubberCapacitance=inf  Measurements=None
  Three-Phase Breaker6 : spsThreePhaseBreakerLib/Three-Phase Breaker  InitialState=closed  SwitchA=on  SwitchB=on  SwitchC=on  SwitchTimes=[10000000000]  External=off  BreakerResistance=0.00001  SnubberResistance=1e16  SnubberCapacitance=inf  Measurements=None
  Three-Phase Source : spsThreePhaseSourceLib/Three-Phase Source  InternalConnection=Yg  VoltagePhases=off  Voltage=(150420)*1.01398  PhaseAngle=-26.0476  Voltage_phases=[25e3 25e3 25e3]/sqrt(3)  PhaseAngles_phases=[0 -120 +120]  Frequency=60  NonIdealSource=on  SpecifyImpedance=off  Resistance=0.8929  Inductance=16.58e-3  ShortCircuitLevel=100e6  BaseVoltage=150.42e3  XRratio=7  BusType=PQ  Pref=0  Qref=30144000  Prefabc=[10e3, 10e3, 10e3]  Qrefabc=[0, 0, 0]  Qmin=-inf  Qmax=inf
  Three-Phase Source1 : spsThreePhaseSourceLib/Three-Phase Source  InternalConnection=Yg  VoltagePhases=off  Voltage=(147660)*1.00332  PhaseAngle=-26.1108  Voltage_phases=[25e3 25e3 25e3]/sqrt(3)  PhaseAngles_phases=[0 -120 +120]  Frequency=60  NonIdealSource=on  SpecifyImpedance=off  Resistance=0.8929  Inductance=16.58e-3  ShortCircuitLevel=100e6  BaseVoltage=147.66e3  XRratio=7  BusType=PQ  Pref=0  Qref=25276000  Prefabc=[10e3, 10e3, 10e3]  Qrefabc=[0, 0, 0]  Qmin=-inf  Qmax=inf
  Tie-Line Power Flow Sensor : Subsystem
      mask Display: image('$imagefile'); % Use "Edit Image" on toolstrip to change.
  To Workspace : ToWorkspace  VariableName=average_frequency_14_bus  SaveFormat=Timeseries  SampleTime=5e-5
  To Workspace1 : ToWorkspace  VariableName=transmission_line_voltage_14_bus  SaveFormat=Timeseries  SampleTime=5e-5
  To Workspace2 : ToWorkspace  VariableName=average_electrical_power_14_bus  SaveFormat=Timeseries  SampleTime=5e-5
  To Workspace3 : ToWorkspace  VariableName=voltage_angle_14_bus  SaveFormat=Timeseries  SampleTime=5e-5
  Total Harmonic Distortion : eeTotalHarmonicDistorsion/Total Harmonic Distortion  f=60  Ts=-1
      settings: SourceProductBaseCode=PS
  Turbine & Regulators M1 : Subsystem
      settings: PortSchema="{\"entries\":[{\"content\":{\"sides\":[{\"content\":{\"connectorIds\":[\"In1\",\"In2\"]},\"type\":\"ConnectorPlacement.EquallySpacedRectSide\",\"uuid\":\"179db3d5-b74c-4029-b588-072e3e481cea\"},{\"content\":{\"connectorIds\":[\"Out1\",\"In3\",\"Out2\",\"In4\",\"In5\"],\"side\":\"RIGHT\"},\"type\":\"ConnectorPlacement.EquallySpacedRectSide\",\"uuid\":\"30eca1c0-2026-478c-b07c-22fdd6324b2d\"},{\"content\":{\"connectorIds\":[],\"side\":\"TOP\"},\"type\":\"ConnectorPlacement.EquallySpacedRectSide\",\"uuid\":\"6c0565ca-46be-436e-b0e3-ae415eccc3b3\"}]},\"type\":\"ConnectorPlacement.EquallySpacedConnector\",\"uuid\":\"ea6df20e-2d87-46be-9861-8a42788d452f\"}],\"packageUris\":[\"http://schema.mathworks.com/mf0/Connector/R2020b\"],\"version\":\"1.0\"}"
  Turbine & Regulators M2 : Subsystem
      settings: PortSchema="{\"entries\":[{\"content\":{\"sides\":[{\"content\":{\"connectorIds\":[\"In1\",\"In2\",\"In3\"]},\"type\":\"ConnectorPlacement.EquallySpacedRectSide\",\"uuid\":\"7c336a41-84fd-4750-b337-761c590caed7\"},{\"content\":{\"connectorIds\":[\"Out1\",\"In4\",\"In5\",\"Out2\"],\"side\":\"RIGHT\"},\"type\":\"ConnectorPlacement.EquallySpacedRectSide\",\"uuid\":\"226eeb8e-9788-46cb-8233-fba7aeee5eb3\"},{\"content\":{\"connectorIds\":[],\"side\":\"TOP\"},\"type\":\"ConnectorPlacement.EquallySpacedRectSide\",\"uuid\":\"40e33e3a-e732-4755-8b28-e93c478871b8\"}]},\"type\":\"ConnectorPlacement.EquallySpacedConnector\",\"uuid\":\"84b04018-97dd-4be5-b098-b2c811f719d7\"}],\"packageUris\":[\"http://schema.mathworks.com/mf0/Connector/R2020b\"],\"version\":\"1.0\"}"
  Turbine & Regulators M3 : Subsystem
      settings: PortSchema="{\"entries\":[{\"content\":{\"sides\":[{\"content\":{\"connectorIds\":[\"In1\",\"In2\"]},\"type\":\"ConnectorPlacement.EquallySpacedRectSide\",\"uuid\":\"179db3d5-b74c-4029-b588-072e3e481cea\"},{\"content\":{\"connectorIds\":[\"Out1\",\"In3\",\"In4\",\"Out2\"],\"side\":\"RIGHT\"},\"type\":\"ConnectorPlacement.EquallySpacedRectSide\",\"uuid\":\"30eca1c0-2026-478c-b07c-22fdd6324b2d\"},{\"content\":{\"connectorIds\":[],\"side\":\"TOP\"},\"type\":\"ConnectorPlacement.EquallySpacedRectSide\",\"uuid\":\"6c0565ca-46be-436e-b0e3-ae415eccc3b3\"}]},\"type\":\"ConnectorPlacement.EquallySpacedConnector\",\"uuid\":\"ea6df20e-2d87-46be-9861-8a42788d452f\"}],\"packageUris\":[\"http://schema.mathworks.com/mf0/Connector/R2020b\"],\"version\":\"1.0\"}"
  Vref1 1 : Constant  Value=1.6922
  Vref2 : Constant
  powergui : spspowerguiLib/powergui  Priority=1  SimulationMode=Discrete  SampleTime=5e-5  frequency=60  Iterations=2000  frequencyindice=60  Pbase=100e6  ErrMax=0.0001  UnitsV=kV  UnitsW=MW  buscounter=0  FunctionMessages=off  echomessages=off  EnableUseOfTLC=off  CurrentSourceSwitches=off  DisableSnubberDevices=off  DisableRonSwitches=off  DisableVfSwitches=off  DisplayEquations=off  AutomaticDiscreteSolvers=off  SolverType=Tustin/Backward Euler (TBE)  Interpol=off  ExternalGateDelay=off  methode=off  Ts=100  x0status=blocks  SPID=on  SwTol=0  HookPort=off  NonlinearTolerance=1e-4  nMaxIteration=100  ContinueOnMaxIteration=off  RestoreLinks=warning  ResistiveCurrentMeasurement=off  Frange=[0:2:500]  Ylog=off  Xlog=on  ShowGrid=off  save=off  variable=ZData  structure=0  ZoomFFT=off  StartTime=0.0  cycles=1  DisplayStyle=1  fundamental=60  FreqAxis=off  MaxFrequency=1000  frequencyindicesteady=1  RmsSteady=1  display=off
  tag scope: PSS=global
  wires:
  Total Harmonic Distortion/1 -> DEFENDER REWARD FUNCTION/5(DATHD), Scope21/1
  "PMU (PLL-Based, Positive-Sequence)"/2 -> Mux1/5, Mux1/4, DEFENDER REWARD FUNCTION/4(DAR), To Workspace3/1, Scope16/1
  Matrix Multiply8/1 -> Rate Transition4/1, Synchronous Machine pu Standard2/1
  Turbine & Regulators M3/2(Vf) -> Matrix Multiply7/2
  NOT3/1 -> Matrix Multiply8/1, Matrix Multiply7/1
  Matrix Multiply7/1 -> Scope15/1, Rate Transition5/1, Synchronous Machine pu Standard2/2
  Matrix Multiply6/1 -> Bus Creator/2, Synchronous Machine pu Standard/2
  Turbine & Regulators M2/2(Vf) -> Matrix Multiply6/2
  Turbine & Regulators M2/1(Pm) -> Matrix Multiply5/2
  Matrix Multiply5/1 -> Synchronous Machine pu Standard/1, Bus Creator/1, Scope14/1
  NOT1/1 -> Matrix Multiply5/1, Matrix Multiply6/1
  Matrix Multiply4/1 -> Rate Transition2/1, Synchronous Machine pu Standard1/1
  Turbine & Regulators M1/1(Pm) -> Matrix Multiply4/2
  Matrix Multiply3/1 -> Scope13/1, Rate Transition3/1, Synchronous Machine pu Standard1/2
  Turbine & Regulators M1/2(Vf) -> Matrix Multiply3/2
  NOT2/1 -> NOT/1, Matrix Multiply4/1, Matrix Multiply3/1
  Fcn2/1 -> Mux1/2, Compare To Constant3/1, Compare To Constant2/1, Turbine & Regulators M1/5(Inport), Scope6/1
  PID Controller2/1 -> Sum1/2, Sum2/2
  PID Controller1/1 -> Sum/2
  NOT/1 -> Scope10/1, Three-Phase Breaker/1
  ? -> ?
  Three-Phase V-I Measurement9/1 -> Scope47/1
  Three-Phase V-I Measurement5/1 -> Scope7/1
  Three-Phase V-I Measurement6/2 -> Scope/1
  Constant1/1 -> Sum1/1
  MATLAB Function2/1(y) -> Scope19/1
  Kalman Filter1/1 -> Matrix Multiply1/2
  Sum/1 -> Turbine & Regulators M3/2(Pref)
  Bus Selector3/1 -> PID Controller2/1, DEFENDER REWARD FUNCTION/2(DAF2), Fcn2/1  "<Rotor speed deviation  dw (pu)>"
  Synchronous Machine pu Standard1/1 -> Subtract1/1, Kalman Filter1/2, Bus Selector3/1, Turbine & Regulators M1/1(m)
  Rate Transition5/1 -> Bus Creator2/2
  Synchronous Machine pu Standard2/1 -> Subtract2/1, Kalman Filter2/2, Bus Selector1/1, Turbine & Regulators M3/1(m)
  Subtract1/1 -> MATLAB Function1/1(u)
  Turbine & Regulators M3/1(Pm) -> Matrix Multiply8/2
  Fcn3/1 -> DEFENDER REWARD FUNCTION/1(DAF1), Mux1/1, Compare To Constant1/1, Compare To Constant/1, Turbine & Regulators M2/5(Inport), Scope4/1
  Bus Selector2/1 -> Fcn3/1  "<Rotor speed deviation  dw (pu)>"
  Constant11/1 -> Kalman Filter2/4
  Vref2/1 -> Turbine & Regulators M2/3(Vref)
  Constant9/1 -> Matrix Multiply1/1
  Constant6/1 -> Kalman Filter1/3
  Matrix Multiply2/1 -> Subtract2/2
  Constant12/1 -> Kalman Filter2/5
  Subsystem/1(Generic) -> PSS selector/1
  PSS selector1/1 -> [PSS]
  Bus Creator/1 -> Kalman Filter/1
  Kalman Filter/1 -> Matrix Multiply/2
  Three-Phase V-I Measurement2/2 -> Scope11/1
  Subsystem/3(No PSS) -> PSS selector1/2
  Constant3/1 -> Kalman Filter/4
  Constant/1 -> Kalman Filter/3
  Bus Selector1/1 -> PID Controller1/1, Fcn1/1  "<Rotor speed deviation  dw (pu)>"
  Synchronous Machine pu Standard/1 -> Bus Selector2/1, Kalman Filter/2, Subtract/1, Turbine & Regulators M2/1(m)
  Constant2/1 -> Sum/1
  Constant8/1 -> Kalman Filter1/5
  Constant7/1 -> Kalman Filter1/4
  Bus Selector1/2 -> Scope3/1, Total Harmonic Distortion/1, Display5/1  "<Electrical power  Pe (pu)>"
  Kalman Filter2/1 -> Matrix Multiply2/2
  Constant13/1 -> Matrix Multiply2/1
  Constant4/1 -> Kalman Filter/5
  Three-Phase V-I Measurement2/1 -> "PMU (PLL-Based, Positive-Sequence)"/1, To Workspace1/1, Scope24/1
  Matrix Multiply/1 -> Subtract/2
  Rate Transition4/1 -> Bus Creator2/1
  MATLAB Function/1(y) -> Scope1/1
  PSS selector/1 -> PSS selector1/1
  Constant10/1 -> Kalman Filter2/3
  Sum2/1 -> Turbine & Regulators M2/2(Pref)
  Rate Transition3/1 -> Bus Creator1/2
  Matrix Multiply1/1 -> Subtract1/2
  Bus Creator2/1 -> Kalman Filter2/1
  Fcn1/1 -> Turbine & Regulators M3/4(Inport), DEFENDER REWARD FUNCTION/3(DAF3), Mux1/3, Compare To Constant5/1, Compare To Constant4/1, To Workspace/1, Scope2/1
  Bus Selector2/2 -> Display1/1, Scope5/1, To Workspace2/1  "<Electrical power  Pe (pu)>"
  Constant5/1 -> Matrix Multiply/1
  Bus Creator1/1 -> Kalman Filter1/1
  Three-Phase V-I Measurement8/1 -> Scope18/1
  Subsystem/2(Multiband) -> PSS selector/2
  Subtract2/1 -> MATLAB Function2/1(u)
  Three-Phase V-I Measurement4/1 -> Scope20/1
  Rate Transition2/1 -> Bus Creator1/1
  Subtract/1 -> MATLAB Function/1(u)
  MATLAB Function1/1(y) -> Scope8/1
  Three-Phase V-I Measurement7/1 -> Scope17/1
  Sum1/1 -> Turbine & Regulators M1/2(Pref)
  Vref1 1/1 -> Sum2/1
  Bus Selector3/2 -> Scope9/1  "<Electrical power  Pe (pu)>"
  Three-Phase V-I Measurement3/1 -> Scope12/1
  Compare To Constant1/1 -> OR/1
  Compare To Constant/1 -> OR/2
  Compare To Constant2/1 -> OR1/2
  Compare To Constant3/1 -> OR1/1
  Compare To Constant4/1 -> OR2/1
  Compare To Constant5/1 -> OR2/2
  OR/1 -> NOT1/1
  OR1/1 -> NOT2/1
  OR2/1 -> NOT3/1
  RL Agent/1 -> Demux1/1
  Mux1/1 -> RL Agent/1
  DEFENDER REWARD FUNCTION/1(REWARD_DEFENDER) -> RL Agent/2
  Constant14/1 -> RL Agent/3
  Demux1/1 -> Turbine & Regulators M2/4(In4)
  Demux1/2 -> Turbine & Regulators M1/3(In3)
  Demux1/3 -> Turbine & Regulators M3/3(In3)
  Demux1/4 -> Turbine & Regulators M1/4(In4)
  connections:
  Bus_13/LConn3 -- Three-Phase Series RLC Load8/LConn1
  Bus_13/LConn2 -- Three-Phase Series RLC Load8/LConn2
  Bus_13/LConn1 -- Three-Phase Series RLC Load8/LConn3
  Three-Phase Breaker6/RConn3 -- Bus_10/LConn3
  Three-Phase Breaker6/RConn2 -- Bus_10/LConn2
  Three-Phase Breaker6/RConn1 -- Bus_10/LConn1
  Three-Phase Breaker6/LConn1 -- Three-Phase Series RLC Load5/LConn1
  Three-Phase Breaker6/LConn2 -- Three-Phase Series RLC Load5/LConn2
  Three-Phase Breaker6/LConn3 -- Three-Phase Series RLC Load5/LConn3
  Three-Phase Series RLC Load2/LConn1 -- Bus_4/RConn10
  Three-Phase Series RLC Load2/LConn3 -- Bus_4/RConn12
  Bus_4/RConn11 -- Three-Phase Series RLC Load2/LConn2
  Three-Phase Breaker4/LConn3 -- Three-Phase Series RLC Load3/LConn3
  Three-Phase Breaker4/RConn3 -- Bus_5/LConn1
  Three-Phase Breaker4/LConn2 -- Three-Phase Series RLC Load3/LConn2
  Three-Phase Breaker4/RConn2 -- Bus_5/LConn2
  Three-Phase Breaker4/LConn1 -- Three-Phase Series RLC Load3/LConn1
  Three-Phase Breaker4/RConn1 -- Bus_5/LConn3
  Three-Phase Series RLC Load4/LConn1 -- Three-Phase Breaker3/LConn1
  Three-Phase Breaker3/RConn1 -- Bus_6/RConn7
  Three-Phase Series RLC Load4/LConn2 -- Three-Phase Breaker3/LConn2
  Bus_6/RConn12 -- Three-Phase Breaker3/RConn2
  Three-Phase Breaker3/LConn3 -- Three-Phase Series RLC Load4/LConn3
  Three-Phase Breaker3/RConn3 -- Bus_6/RConn13
  Three-Phase Breaker2/LConn3 -- Three-Phase Series RLC Load7/LConn3
  Bus_12/LConn3 -- Three-Phase Breaker2/RConn3
  Three-Phase Breaker2/LConn2 -- Three-Phase Series RLC Load7/LConn2
  Bus_12/LConn2 -- Three-Phase Breaker2/RConn2
  Three-Phase Breaker2/LConn1 -- Three-Phase Series RLC Load7/LConn1
  Bus_12/LConn1 -- Three-Phase Breaker2/RConn1
  Three-Phase Breaker1/LConn3 -- Three-Phase Series RLC Load9/LConn3
  Bus_9/RConn10 -- Three-Phase Breaker1/RConn3
  Three-Phase Breaker1/LConn2 -- Three-Phase Series RLC Load9/LConn2
  Three-Phase Breaker1/RConn2 -- Bus_9/RConn11
  Three-Phase Breaker1/LConn1 -- Three-Phase Series RLC Load9/LConn1
  Three-Phase Breaker1/RConn1 -- Bus_9/RConn12
  Three-Phase Series RLC Load14/LConn3 -- Three-Phase Breaker/RConn3
  Three-Phase Series RLC Load14/LConn2 -- Three-Phase Breaker/RConn2
  Three-Phase Series RLC Load14/LConn1 -- Three-Phase Breaker/RConn1
  Subsystem2/LConn1 -- Three-Phase Breaker/LConn1 -- Bus_3/RConn4
  Bus_12/RConn1 -- Three-Phase PI Section Line14/LConn1
  Bus_9/LConn3 -- Three-Phase PI Section Line19/RConn3
  Three-Phase Source/RConn1 -- Three-Phase Transformer (Two Windings)4/LConn1
  Bus_1/LConn3 -- Three-Phase Transformer (Two Windings)/RConn1
  Bus_12/RConn2 -- Three-Phase PI Section Line14/LConn2
  Bus_14/LConn3 -- Three-Phase Series RLC Load12/LConn3
  Three-Phase Transformer (Two Windings)2/LConn3 -- Three-Phase Source1/RConn3
  Three-Phase PI Section Line8/LConn3 -- Bus_7/RConn6
  Three-Phase PI Section Line13/LConn2 -- Bus_6/LConn4
  Bus_6/LConn1 -- Three-Phase Transformer (Two Windings)2/RConn1
  Three-Phase PI Section Line14/RConn1 -- Bus_6/RConn1
  Bus_9/LConn5 -- Three-Phase Series RLC Load11/LConn2
  Three-Phase Transformer (Two Windings)3/RConn1 -- Bus_3/RConn7
  Three-Phase PI Section Line2/LConn1 -- Bus_2/LConn6
  Bus_9/RConn3 -- Three-Phase PI Section Line11/RConn3
  Three-Phase Transformer (Two Windings)4/RConn2 -- Three-Phase V-I Measurement/RConn2
  Bus_11/LConn3 -- Three-Phase Series RLC Load6/LConn3
  Bus_5/RConn6 -- Three-Phase PI Section Line2/RConn1
  Three-Phase PI Section Line19/LConn1 -- Bus_14/RConn4
  Bus_7/RConn3 -- Three-Phase PI Section Line9/RConn3
  Three-Phase PI Section Line10/LConn2 -- Bus_9/RConn5
  Bus_13/RConn2 -- Three-Phase PI Section Line15/RConn2
  Bus_5/RConn2 -- Three-Phase PI Section Line1/RConn2
  Bus_4/LConn1 -- Three-Phase PI Section Line10/RConn1
  Bus_4/LConn2 -- Three-Phase PI Section Line10/RConn2
  Three-Phase PI Section Line7/RConn1 -- Bus_4/LConn4
  Three-Phase PI Section Line3/LConn2 -- Bus_5/RConn8
  Bus_4/RConn1 -- Three-Phase PI Section Line3/RConn1
  Three-Phase PI Section Line13/LConn3 -- Bus_6/LConn5
  Bus_4/RConn3 -- Three-Phase PI Section Line3/RConn3
  Bus_7/RConn1 -- Three-Phase PI Section Line9/RConn1
  Three-Phase PI Section Line7/LConn2 -- Bus_7/LConn2
  Three-Phase V-I Measurement/LConn2 -- Three-Phase PI Section Line8/RConn2
  Three-Phase PI Section Line11/LConn2 -- Bus_10/RConn5
  Three-Phase Transformer (Two Windings)3/RConn2 -- Bus_3/RConn8
  Three-Phase PI Section Line12/LConn1 -- Bus_11/RConn6
  Three-Phase PI Section Line15/LConn3 -- Bus_12/RConn4
  Three-Phase PI Section Line7/RConn2 -- Bus_4/LConn5
  Bus_6/RConn10 -- Three-Phase PI Section Line17/LConn1
  Bus_12/RConn3 -- Three-Phase PI Section Line14/LConn3
  Three-Phase PI Section Line16/LConn1 -- Bus_13/RConn4
  Bus_6/RConn9 -- Three-Phase PI Section Line16/RConn3
  Three-Phase PI Section Line6/RConn3 -- Bus_3/LConn3
  Three-Phase PI Section Line8/LConn2 -- Bus_7/RConn5
  Bus_7/RConn2 -- Three-Phase PI Section Line9/RConn2
  Three-Phase PI Section Line10/LConn3 -- Bus_9/RConn6
  Bus_13/RConn3 -- Three-Phase PI Section Line15/RConn3
  Three-Phase Series RLC Load12/LConn2 -- Bus_14/LConn2
  Bus_10/RConn1 -- Three-Phase PI Section Line12/RConn1
  Bus_4/RConn2 -- Three-Phase PI Section Line3/RConn2
  Bus_2/LConn3 -- Three-Phase PI Section Line/RConn3
  Three-Phase PI Section Line3/LConn1 -- Bus_5/RConn9
  Three-Phase PI Section Line8/LConn1 -- Bus_7/RConn4
  Three-Phase PI Section Line2/LConn3 -- Bus_2/LConn4
  Bus_1/RConn1 -- Three-Phase PI Section Line/LConn1
  Bus_6/LConn3 -- Three-Phase Transformer (Two Windings)2/RConn2
  Bus_4/RConn9 -- Three-Phase PI Section Line6/LConn3
  Three-Phase PI Section Line7/LConn1 -- Bus_7/LConn1
  Three-Phase PI Section Line2/LConn2 -- Bus_2/LConn5
  Bus_6/RConn6 -- Three-Phase PI Section Line17/LConn3
  Bus_6/RConn5 -- Three-Phase PI Section Line17/LConn2
  Three-Phase PI Section Line12/LConn3 -- Bus_11/RConn4
  Bus_5/RConn4 -- Three-Phase PI Section Line2/RConn3
  Bus_6/RConn4 -- Three-Phase PI Section Line16/RConn1
  Three-Phase Transformer (Two Windings)3/RConn3 -- Bus_3/RConn9
  Bus_4/RConn8 -- Three-Phase PI Section Line6/LConn2
  Three-Phase PI Section Line7/RConn3 -- Bus_4/LConn6
  Three-Phase Transformer (Two Windings)1/RConn2 -- Bus_2/RConn8
  Three-Phase PI Section Line14/RConn3 -- Bus_6/RConn3
  Three-Phase PI Section Line15/LConn1 -- Bus_12/RConn6
  Bus_9/LConn4 -- Three-Phase Series RLC Load11/LConn1
  Three-Phase PI Section Line15/LConn2 -- Bus_12/RConn5
  Three-Phase PI Section Line11/LConn1 -- Bus_10/RConn6
  Three-Phase PI Section Line9/LConn2 -- Bus_9/RConn8
  Three-Phase PI Section Line7/LConn3 -- Bus_7/LConn3
  Three-Phase PI Section Line13/RConn3 -- Bus_5/LConn6
  Three-Phase PI Section Line16/LConn3 -- Bus_13/RConn6
  Bus_9/RConn1 -- Three-Phase PI Section Line11/RConn1
  Three-Phase PI Section Line19/LConn3 -- Bus_14/RConn6
  Three-Phase PI Section Line11/LConn3 -- Bus_10/RConn4
  Bus_1/LConn1 -- Three-Phase Transformer (Two Windings)/RConn3
  Three-Phase PI Section Line8/RConn1 -- Three-Phase V-I Measurement/LConn1
  Bus_1/RConn5 -- Three-Phase PI Section Line1/LConn2
  Three-Phase Transformer (Two Windings)2/LConn2 -- Three-Phase Source1/RConn2
  Bus_5/RConn3 -- Three-Phase PI Section Line1/RConn3
  Bus_5/RConn5 -- Three-Phase PI Section Line2/RConn2
  Three-Phase PI Section Line10/LConn1 -- Bus_9/RConn4
  Three-Phase PI Section Line9/LConn3 -- Bus_9/RConn9
  Bus_9/LConn1 -- Three-Phase PI Section Line19/RConn1
  Bus_10/RConn3 -- Three-Phase PI Section Line12/RConn3
  Bus_1/RConn4 -- Three-Phase PI Section Line1/LConn3
  Bus_5/RConn1 -- Three-Phase PI Section Line1/RConn1
  Bus_13/RConn1 -- Three-Phase PI Section Line15/RConn1
  Bus_1/LConn2 -- Three-Phase Transformer (Two Windings)/RConn2
  Bus_2/LConn2 -- Three-Phase PI Section Line/RConn2
  Bus_11/LConn1 -- Three-Phase Series RLC Load6/LConn1
  Three-Phase PI Section Line19/LConn2 -- Bus_14/RConn5
  Three-Phase Source/RConn2 -- Three-Phase Transformer (Two Windings)4/LConn2
  Three-Phase PI Section Line13/LConn1 -- Bus_6/RConn11
  Bus_2/LConn1 -- Three-Phase PI Section Line/RConn1
  Three-Phase PI Section Line13/RConn1 -- Bus_5/LConn4
  Bus_9/LConn6 -- Three-Phase Series RLC Load11/LConn3
  Three-Phase PI Section Line8/RConn3 -- Three-Phase V-I Measurement/LConn3
  Bus_1/RConn3 -- Three-Phase PI Section Line/LConn3
  Three-Phase Transformer (Two Windings)2/LConn1 -- Three-Phase Source1/RConn1
  Bus_10/RConn2 -- Three-Phase PI Section Line12/RConn2
  Three-Phase Transformer (Two Windings)4/RConn3 -- Three-Phase V-I Measurement/RConn3
  Bus_14/LConn1 -- Three-Phase Series RLC Load12/LConn1
  Bus_9/RConn2 -- Three-Phase PI Section Line11/RConn2
  Three-Phase PI Section Line6/RConn1 -- Bus_3/LConn1
  Three-Phase Source/RConn3 -- Three-Phase Transformer (Two Windings)4/LConn3
  Bus_6/RConn8 -- Three-Phase PI Section Line16/RConn2
  Bus_4/RConn7 -- Three-Phase PI Section Line6/LConn1
  Bus_1/RConn2 -- Three-Phase PI Section Line/LConn2
  Three-Phase Transformer (Two Windings)1/RConn1 -- Bus_2/RConn7
  Three-Phase PI Section Line14/RConn2 -- Bus_6/RConn2
  Three-Phase Transformer (Two Windings)4/RConn1 -- Three-Phase V-I Measurement/RConn1
  Bus_11/RConn1 -- Three-Phase PI Section Line17/RConn1
  Bus_11/RConn2 -- Three-Phase PI Section Line17/RConn2
  Bus_4/LConn3 -- Three-Phase PI Section Line10/RConn3
  Three-Phase PI Section Line3/LConn3 -- Bus_5/RConn7
  Bus_1/RConn6 -- Three-Phase PI Section Line1/LConn1
  Bus_11/RConn3 -- Three-Phase PI Section Line17/RConn3
  Bus_6/LConn2 -- Three-Phase Transformer (Two Windings)2/RConn3
  Three-Phase PI Section Line13/RConn2 -- Bus_5/LConn5
  Three-Phase PI Section Line6/RConn2 -- Bus_3/LConn2
  Three-Phase PI Section Line16/LConn2 -- Bus_13/RConn5
  Bus_2/RConn9 -- Three-Phase Transformer (Two Windings)1/RConn3
  Three-Phase PI Section Line12/LConn2 -- Bus_11/RConn5
  Bus_9/LConn2 -- Three-Phase PI Section Line19/RConn2
  Three-Phase PI Section Line9/LConn1 -- Bus_9/RConn7
  Three-Phase Series RLC Load6/LConn2 -- Bus_11/LConn2
  Three-Phase PI Section Line18/LConn1 -- Bus_13/RConn9 -- Three-Phase V-I Measurement7/LConn1
  Three-Phase PI Section Line5/LConn2 -- Three-Phase V-I Measurement2/LConn2 -- Bus_2/RConn11
  Bus_3/RConn2 -- Three-Phase V-I Measurement4/LConn2 -- Three-Phase PI Section Line5/RConn2
  Three-Phase Transformer (Two Windings)3/LConn3 -- Three-Phase V-I Measurement1/LConn3 -- Synchronous Machine pu Standard2/RConn3 -- Three-Phase Parallel RLC Load2/LConn3
  Three-Phase PI Section Line5/LConn1 -- Three-Phase V-I Measurement2/LConn1 -- Bus_2/RConn12
  Bus_2/RConn5 -- Three-Phase Series RLC Load10/LConn2
  Bus_14/RConn3 -- Three-Phase V-I Measurement8/LConn3 -- Three-Phase PI Section Line18/RConn3
  Three-Phase V-I Measurement3/LConn2 -- Synchronous Machine pu Standard1/RConn2 -- Three-Phase Transformer (Two Windings)1/LConn2 -- Three-Phase Parallel RLC Load1/LConn2
  Bus_2/RConn6 -- Three-Phase Series RLC Load10/LConn3
  Bus_4/RConn5 -- Three-Phase V-I Measurement6/LConn2 -- Three-Phase PI Section Line4/RConn2
  Bus_14/RConn2 -- Three-Phase V-I Measurement8/LConn2 -- Three-Phase PI Section Line18/RConn2
  Subsystem2/LConn2 -- Three-Phase Breaker/LConn2 -- Bus_3/RConn5
  Bus_4/RConn4 -- Three-Phase V-I Measurement6/LConn1 -- Three-Phase PI Section Line4/RConn1
  Three-Phase Parallel RLC Load2/LConn1 -- Synchronous Machine pu Standard2/RConn1 -- Three-Phase V-I Measurement1/LConn1 -- Three-Phase Transformer (Two Windings)3/LConn1
  Three-Phase PI Section Line5/LConn3 -- Three-Phase V-I Measurement2/LConn3 -- Bus_2/RConn10
  Three-Phase Transformer (Two Windings)1/LConn1 -- Three-Phase Parallel RLC Load1/LConn1 -- Three-Phase V-I Measurement3/LConn1 -- Synchronous Machine pu Standard1/RConn1
  Three-Phase PI Section Line18/LConn3 -- Three-Phase V-I Measurement7/LConn3 -- Bus_13/RConn7
  Bus_3/RConn1 -- Three-Phase V-I Measurement4/LConn1 -- Three-Phase PI Section Line5/RConn1
  Three-Phase Transformer (Two Windings)1/LConn3 -- Three-Phase V-I Measurement3/LConn3 -- Synchronous Machine pu Standard1/RConn3 -- Three-Phase Parallel RLC Load1/LConn3
  Bus_14/RConn1 -- Three-Phase V-I Measurement8/LConn1 -- Three-Phase PI Section Line18/RConn1
  Bus_2/RConn3 -- Three-Phase Series RLC Load10/LConn1
  Subsystem2/LConn3 -- Three-Phase Breaker/LConn3 -- Bus_3/RConn6
  Bus_3/RConn3 -- Three-Phase V-I Measurement4/LConn3 -- Three-Phase PI Section Line5/RConn3
  Three-Phase PI Section Line4/LConn3 -- Three-Phase V-I Measurement5/LConn3 -- Bus_2/LConn9
  Synchronous Machine pu Standard/RConn1 -- Three-Phase Transformer (Two Windings)/LConn1 -- Tie-Line Power Flow Sensor/LConn1 -- Three-Phase Parallel RLC Load3/LConn1 -- Three-Phase V-I Measurement9/LConn1
  Three-Phase V-I Measurement1/LConn2 -- Synchronous Machine pu Standard2/RConn2 -- Three-Phase Transformer (Two Windings)3/LConn2 -- Three-Phase Parallel RLC Load2/LConn2
  Synchronous Machine pu Standard/RConn2 -- Three-Phase Transformer (Two Windings)/LConn2 -- Tie-Line Power Flow Sensor/LConn2 -- Three-Phase Parallel RLC Load3/LConn2 -- Three-Phase V-I Measurement9/LConn2
  Three-Phase PI Section Line18/LConn2 -- Three-Phase V-I Measurement7/LConn2 -- Bus_13/RConn8
  Bus_4/RConn6 -- Three-Phase V-I Measurement6/LConn3 -- Three-Phase PI Section Line4/RConn3
  Three-Phase PI Section Line4/LConn1 -- Three-Phase V-I Measurement5/LConn1 -- Bus_2/LConn7
  Three-Phase V-I Measurement9/LConn3 -- Synchronous Machine pu Standard/RConn3 -- Three-Phase Transformer (Two Windings)/LConn3 -- Tie-Line Power Flow Sensor/LConn3 -- Three-Phase Parallel RLC Load3/LConn3
  Three-Phase PI Section Line4/LConn2 -- Three-Phase V-I Measurement5/LConn2 -- Bus_2/LConn8
